simulink model "RFB_parasitic_method"  (R2019b)
settings: Solver=VariableStepAuto  StartTime=0.0  StopTime=10.0  RelTol=1e-3
libraries: dspxfrm3 x2, cstblocks x1, simulink_extras x1
settings Model: Creator=rshousha  LastModifiedBy=jwai
settings DataIOCC: ReturnWorkspaceOutputs=off
settings DebuggingCC: ArithmeticOperatorsInVariantConditions=warning
settings SFSimCC: CustomCodeUndefinedFunction=UseInterfaceOnly

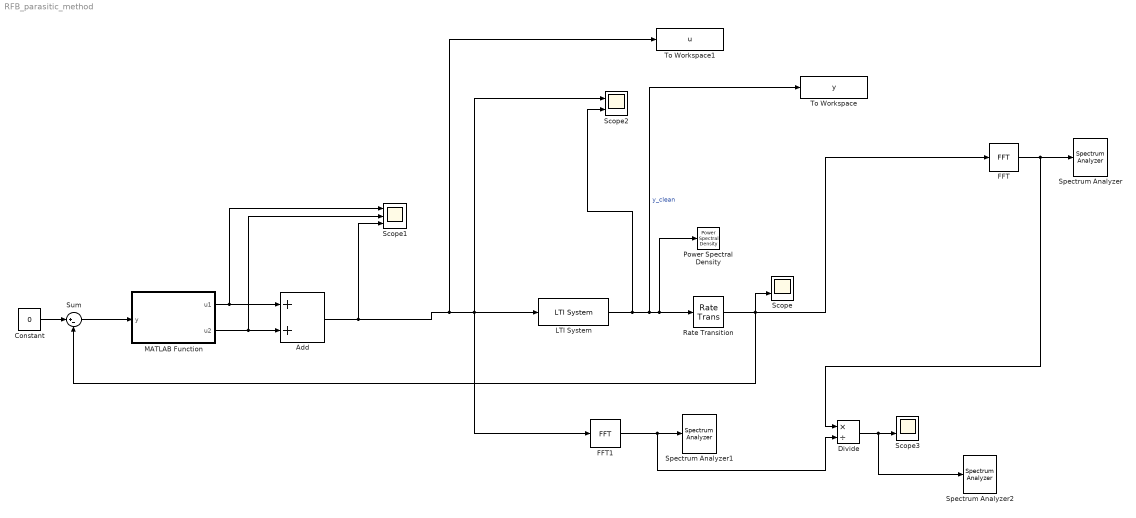
== system RFB_parasitic_method ==
  Add : Sum
  Constant : Constant  Value=0
  Divide : Product  Inputs=*/
  FFT : dspxfrm3/FFT  FFTImplementation=Auto  CompMethod=Table lookup  TableOpt=NEW  TableOptActive=Speed  BitRevOrder=off  Normalize=off  InheritFFTLength=on  FFTLength=64  WrapInput=on  roundingMode=Floor  overflowMode=off  firstCoeffDataTypeStr=Inherit: Same word length as input  firstCoeffLastDataTypeStr=Inherit: Same word length as input  outputMin=[]  outputMax=[]
  FFT1 : dspxfrm3/FFT  FFTImplementation=Auto  CompMethod=Table lookup  TableOpt=NEW  TableOptActive=Speed  BitRevOrder=off  Normalize=off  InheritFFTLength=on  FFTLength=64  WrapInput=on  roundingMode=Floor  overflowMode=off  firstCoeffDataTypeStr=Inherit: Same word length as input  firstCoeffLastDataTypeStr=Inherit: Same word length as input  outputMin=[]  outputMax=[]
  LTI System : cstblocks/LTI System  sys=G_true  IC=[]
  MATLAB Function : MATLAB Function  TreatAsAtomicUnit=on
  Power Spectral Density : simulink_extras/Additional Sinks/Power Spectral Density  npts=128  fftpts=512  HowOften=64  sampleT=0.1
      settings: SourceProductName=Simulink  SourceProductBaseCode=SL
  Rate Transition : RateTransition  OutPortSampleTime=5e-5
  Scope : Scope  NumInputPorts=2
  Scope1 : Scope  NumInputPorts=3
  Scope2 : Scope  NumInputPorts=2
  Scope3 : Scope  NumInputPorts=2
  Spectrum Analyzer : SpectrumAnalyzer
  Spectrum Analyzer1 : SpectrumAnalyzer
  Spectrum Analyzer2 : SpectrumAnalyzer
  Sum : Sum  Inputs=|+-
  To Workspace : ToWorkspace  VariableName=y  SaveFormat=Timeseries  SampleTime=-1
  To Workspace1 : ToWorkspace  VariableName=u  SaveFormat=Timeseries  SampleTime=-1
  wires:
  LTI System/1 -> Scope2/2, To Workspace/1, Power Spectral Density/1, Rate Transition/1  "y_clean"
  Sum/1 -> MATLAB Function/1(y)
  Rate Transition/1 -> FFT/1, Sum/2, Scope/2
  Constant/1 -> Sum/1
  FFT/1 -> Divide/1, Spectrum Analyzer/1
  MATLAB Function/1(u1) -> Scope1/1, Add/1
  MATLAB Function/2(u2) -> Scope1/2, Add/2
  Add/1 -> Scope1/3, To Workspace1/1, Scope2/1, LTI System/1, FFT1/1
  FFT1/1 -> Divide/2, Spectrum Analyzer1/1
  Divide/1 -> Spectrum Analyzer2/1, Scope3/2

== matlab function RFB_parasitic_method/MATLAB Function ==
  data: y input; u1 output; u2 output
function [u1,u2] = parasitic_relay(y)

persistent u1km1 u2km1
h=1;
alpha = 0.2;


if y > 0
    u1 = h;
else
    u1 = -h;
end

if isempty(u1km1)
    u2 = alpha*h;
    u1km1 = u1;
    u2km1 = u2;
else
    if (u1km1 > 0) && (u1 < 0)
        u2 = -alpha*h*sign(u2km1);
    else
        u2 = u2km1;
    end
    u1km1 = u1;
    u2km1 = u2;
end


    
    
end
